simulink model "power_microgrid_v5_battery"  (R2018b)
settings: Solver=ode23tb  StartTime=0.0  StopTime=24*60*60  FixedStep=1/(1000)  MaxStep=60  RelTol=1e-4
PreLoadFcn:
  | load('solar_load_data_24h.mat')
PostLoadFcn:
  | data = xlsread('Domestic_data_all_x3','Sheet1');
  | breakpoints1 = data(2:end,1)'
  | breakpoints2 = data(1,2:end)
  | table_data = data(2:end,2:end)
values from neighbouring files (symbols this model uses):
  SPD_1min = [0 0 0 0 0 0 0 0 0 0 0 0 ... (1441 elements, 1441x1)]    [default_PV_data.mat]
  SPT_1min = [0 60 120 180 240 300 360 420 480 540 600 660 ... (1441 elements, 1441x1)]    [default_PV_data.mat]
libraries: powerlib x155
(part 3 of 5)

== system power_microgrid_v5_battery/House 26 ==
  Clock : Clock
  Complex to Magnitude-Angle : ComplexToMagnitudeAngle  Output=Angle
  Controlled Current Source4 : powerlib/Electrical Sources/Controlled Current Source  Initialize=on  Source_Type=AC  Amplitude=0  Phase=0  Frequency=50  Measurements=None
      settings: SourceProductName=Simscape Electrical
  Gain10 : Gain  Gain=sqrt(2)
  Gain6 : Gain  Gain=-1/230
  Load Data 1-D Lookup Table : Lookup_n-D  NumberOfTableDimensions=1  BreakpointsForDimension1="[0.00\t600.00\t1200.00\t1800.00\t2400.00\t3000.00\t3600.00\t4200.00\t4800.00\t5400.00\t6000.00\t6600.00\t7200.00\t7800.00\t8400.00\t9000.00\t9600.00\t10200.00\t10800.00\t11400.00\t12000.00\t12600.00\t13200.00\t13800.00\t14400.00\t15000.00\t15600.00\t16200.00\t16800.00\t17400.00\t18000.00\t18600.00\t19200.00\t19800.00\t20400.00\t21000.00\t21600.00\t22200.00\t22800.00\t23400.00\t24000.00\t24600.00\t25200.00\t25800.00\t26400.00\t27000.00\t27600.00\t28200.00\t28800.00\t29400.00\t30000.00\t30600.00\t31200.00\t31800.00\t32400.00\t33000.00\t33600.00\t34200.00\t34800.00\t35400.00\t36000.00\t36600.00\t37200.00\t37800.00\t38400.00\t39000.00\t39600.00\t40200.00\t40800.00\t41400.00\t42000.00\t42600.00\t43200.00\t43800.00\t44400.00\t45000.00\t45600.00\t46200.00\t46800.00\t47400.00\t48000.00\t48600.00\t49200.00\t49800.00\t50400.00\t51000.00\t51600.00\t52200.00\t52800.00\t53400.00\t54000.00\t54600.00\t55200.00\t55800.00\t56400.00\t57000.00\t57600.00\t58200.00\t58800.00\t59400.00\t60000.00\t60600.00\t61200.00\t61800.00\t62400.00\t63000.00\t63600.00\t64200.00\t64800.00\t65400.00\t66000.00\t66600.00\t67200.00\t67800.00\t68400.00\t69000.00\t69600.00\t70200.00\t70800.00\t71400.00\t72000.00\t72600.00\t73200.00\t73800.00\t74400.00\t75000.00\t75600.00\t76200.00\t76800.00\t77400.00\t78000.00\t78600.00\t79200.00\t79800.00\t80400.00\t81000.00\t81600.00\t82200.00\t82800.00\t83400.00\t84000.00\t84600.00\t85200.00\t85800.00\t86400.00]"  BeginIndexSearchUsingPreviousIndexResult=on  Table="[176.6\t168.8\t171.0\t162.4\t139.2\t135.7\t136.1\t126.4\t115.3\t119.1\t120.9\t112.9\t108.8\t108.4\t108.6\t115.7\t109.1\t110.1\t104.3\t102.4\t107.1\t108.6\t105.0\t101.7\t101.0\t100.5\t104.1\t105.9\t110.2\t113.1\t112.9\t122.1\t109.2\t120.3\t118.6\t122.6\t124.2\t134.1\t162.8\t189.0\t309.3\t319.3\t364.8\t346.9\t417.0\t276.3\t256.5\t386.4\t343.0\t281.6\t284.9\t297.7\t367.6\t344.5\t340.2\t401.7\t337.5\t290.1\t263.4\t283.0\t256.4\t264.4\t333.9\t339.9\t228.2\t258.4\t286.7\t337.2\t345.7\t283.4\t271.5\t301.9\t315.2\t222.7\t260.5\t314.4\t276.6\t251.0\t286.5\t277.6\t337.1\t293.1\t272.6\t264.0\t234.7\t266.6\t312.4\t300.4\t272.7\t275.3\t328.8\t303.7\t296.9\t271.1\t276.5\t287.6\t336.9\t310.5\t308.1\t352.7\t369.3\t416.5\t395.6\t425.3\t391.6\t343.9\t385.2\t411.7\t419.9\t433.6\t448.9\t437.5\t456.3\t466.2\t475.8\t478.2\t421.9\t455.4\t432.7\t434.7\t414.2\t380.6\t376.3\t380.7\t364.6\t365.6\t376.3\t400.0\t428.4\t382.9\t369.3\t440.8\t388.9\t372.9\t362.3\t328.6\t292.7\t286.7\t266.4\t263.2\t248.0\t239.3\t218.5\t190.8\t176.6]"  InternalRulePriority=Speed  RndMeth=Simplest  InputSameDT=on
  Magnitude-Angle to Complex1 : MagnitudeAngleToComplex
  Snubber3 : powerlib/Elements/Series RLC Branch  LConnTagsString=__new0  RConnTagsString=__new0  BranchType=R  Resistance=1e6  Inductance=1e-3  SetiL0=off  InitialCurrent=0  Capacitance=1e-6  Setx0=off  InitialVoltage=0  Measurements=None
      settings: SourceProductName=Simscape Electrical
  meas cur2 : powerlib/Measurements/Current Measurement  PhasorSimulation=on  OutputType=Complex  PSBequivalent=0
      settings: SourceProductName=Simscape Electrical
  Conn1 : PMIOPort  Side=Left
  Conn2 : PMIOPort  Port=2  Side=Right
  Out1 : Outport
  wires:
  meas cur2/1 -> Out1/1
  Clock/1 -> Load Data 1-D Lookup Table/1
  Magnitude-Angle to Complex1/1 -> Controlled Current Source4/1
  Load Data 1-D Lookup Table/1 -> Gain6/1
  Complex to Magnitude-Angle/1 -> Magnitude-Angle to Complex1/2
  Gain10/1 -> Magnitude-Angle to Complex1/1
  Gain6/1 -> Gain10/1
  [Vsec] -> Complex to Magnitude-Angle/1
  connections:
  Controlled Current Source4/LConn1 -- Conn2/RConn1 -- Snubber3/RConn1
  Controlled Current Source4/RConn1 -- meas cur2/RConn1 -- Snubber3/LConn1
  Conn1/RConn1 -- meas cur2/LConn1

== system power_microgrid_v5_battery/House 27 ==
  Clock : Clock
  Complex to Magnitude-Angle : ComplexToMagnitudeAngle  Output=Angle
  Controlled Current Source4 : powerlib/Electrical Sources/Controlled Current Source  Initialize=on  Source_Type=AC  Amplitude=0  Phase=0  Frequency=50  Measurements=None
      settings: SourceProductName=Simscape Electrical
  Gain10 : Gain  Gain=sqrt(2)
  Gain6 : Gain  Gain=-1/230
  Load Data 1-D Lookup Table : Lookup_n-D  NumberOfTableDimensions=1  BreakpointsForDimension1="[0.00\t600.00\t1200.00\t1800.00\t2400.00\t3000.00\t3600.00\t4200.00\t4800.00\t5400.00\t6000.00\t6600.00\t7200.00\t7800.00\t8400.00\t9000.00\t9600.00\t10200.00\t10800.00\t11400.00\t12000.00\t12600.00\t13200.00\t13800.00\t14400.00\t15000.00\t15600.00\t16200.00\t16800.00\t17400.00\t18000.00\t18600.00\t19200.00\t19800.00\t20400.00\t21000.00\t21600.00\t22200.00\t22800.00\t23400.00\t24000.00\t24600.00\t25200.00\t25800.00\t26400.00\t27000.00\t27600.00\t28200.00\t28800.00\t29400.00\t30000.00\t30600.00\t31200.00\t31800.00\t32400.00\t33000.00\t33600.00\t34200.00\t34800.00\t35400.00\t36000.00\t36600.00\t37200.00\t37800.00\t38400.00\t39000.00\t39600.00\t40200.00\t40800.00\t41400.00\t42000.00\t42600.00\t43200.00\t43800.00\t44400.00\t45000.00\t45600.00\t46200.00\t46800.00\t47400.00\t48000.00\t48600.00\t49200.00\t49800.00\t50400.00\t51000.00\t51600.00\t52200.00\t52800.00\t53400.00\t54000.00\t54600.00\t55200.00\t55800.00\t56400.00\t57000.00\t57600.00\t58200.00\t58800.00\t59400.00\t60000.00\t60600.00\t61200.00\t61800.00\t62400.00\t63000.00\t63600.00\t64200.00\t64800.00\t65400.00\t66000.00\t66600.00\t67200.00\t67800.00\t68400.00\t69000.00\t69600.00\t70200.00\t70800.00\t71400.00\t72000.00\t72600.00\t73200.00\t73800.00\t74400.00\t75000.00\t75600.00\t76200.00\t76800.00\t77400.00\t78000.00\t78600.00\t79200.00\t79800.00\t80400.00\t81000.00\t81600.00\t82200.00\t82800.00\t83400.00\t84000.00\t84600.00\t85200.00\t85800.00\t86400.00]"  BeginIndexSearchUsingPreviousIndexResult=on  Table="[176.6\t168.8\t171.0\t162.4\t139.2\t135.7\t136.1\t126.4\t115.3\t119.1\t120.9\t112.9\t108.8\t108.4\t108.6\t115.7\t109.1\t110.1\t104.3\t102.4\t107.1\t108.6\t105.0\t101.7\t101.0\t100.5\t104.1\t105.9\t110.2\t113.1\t112.9\t122.1\t109.2\t120.3\t118.6\t122.6\t124.2\t134.1\t162.8\t189.0\t309.3\t319.3\t364.8\t346.9\t417.0\t276.3\t256.5\t386.4\t343.0\t281.6\t284.9\t297.7\t367.6\t344.5\t340.2\t401.7\t337.5\t290.1\t263.4\t283.0\t256.4\t264.4\t333.9\t339.9\t228.2\t258.4\t286.7\t337.2\t345.7\t283.4\t271.5\t301.9\t315.2\t222.7\t260.5\t314.4\t276.6\t251.0\t286.5\t277.6\t337.1\t293.1\t272.6\t264.0\t234.7\t266.6\t312.4\t300.4\t272.7\t275.3\t328.8\t303.7\t296.9\t271.1\t276.5\t287.6\t336.9\t310.5\t308.1\t352.7\t369.3\t416.5\t395.6\t425.3\t391.6\t343.9\t385.2\t411.7\t419.9\t433.6\t448.9\t437.5\t456.3\t466.2\t475.8\t478.2\t421.9\t455.4\t432.7\t434.7\t414.2\t380.6\t376.3\t380.7\t364.6\t365.6\t376.3\t400.0\t428.4\t382.9\t369.3\t440.8\t388.9\t372.9\t362.3\t328.6\t292.7\t286.7\t266.4\t263.2\t248.0\t239.3\t218.5\t190.8\t176.6]"  InternalRulePriority=Speed  RndMeth=Simplest  InputSameDT=on
  Magnitude-Angle to Complex1 : MagnitudeAngleToComplex
  Snubber3 : powerlib/Elements/Series RLC Branch  LConnTagsString=__new0  RConnTagsString=__new0  BranchType=R  Resistance=1e6  Inductance=1e-3  SetiL0=off  InitialCurrent=0  Capacitance=1e-6  Setx0=off  InitialVoltage=0  Measurements=None
      settings: SourceProductName=Simscape Electrical
  meas cur2 : powerlib/Measurements/Current Measurement  PhasorSimulation=on  OutputType=Complex  PSBequivalent=0
      settings: SourceProductName=Simscape Electrical
  Conn1 : PMIOPort  Side=Left
  Conn2 : PMIOPort  Port=2  Side=Right
  Out1 : Outport
  wires:
  meas cur2/1 -> Out1/1
  Clock/1 -> Load Data 1-D Lookup Table/1
  Magnitude-Angle to Complex1/1 -> Controlled Current Source4/1
  Load Data 1-D Lookup Table/1 -> Gain6/1
  Complex to Magnitude-Angle/1 -> Magnitude-Angle to Complex1/2
  Gain10/1 -> Magnitude-Angle to Complex1/1
  Gain6/1 -> Gain10/1
  [Vsec] -> Complex to Magnitude-Angle/1
  connections:
  Conn1/RConn1 -- meas cur2/LConn1
  Snubber3/LConn1 -- meas cur2/RConn1 -- Controlled Current Source4/RConn1
  Snubber3/RConn1 -- Controlled Current Source4/LConn1 -- Conn2/RConn1

== system power_microgrid_v5_battery/House 28 ==
  Clock : Clock
  Complex to Magnitude-Angle : ComplexToMagnitudeAngle  Output=Angle
  Controlled Current Source4 : powerlib/Electrical Sources/Controlled Current Source  Initialize=on  Source_Type=AC  Amplitude=0  Phase=0  Frequency=50  Measurements=None
      settings: SourceProductName=Simscape Electrical
  Gain10 : Gain  Gain=sqrt(2)
  Gain6 : Gain  Gain=-1/230
  Load Data 1-D Lookup Table : Lookup_n-D  NumberOfTableDimensions=1  BreakpointsForDimension1="[0.00\t600.00\t1200.00\t1800.00\t2400.00\t3000.00\t3600.00\t4200.00\t4800.00\t5400.00\t6000.00\t6600.00\t7200.00\t7800.00\t8400.00\t9000.00\t9600.00\t10200.00\t10800.00\t11400.00\t12000.00\t12600.00\t13200.00\t13800.00\t14400.00\t15000.00\t15600.00\t16200.00\t16800.00\t17400.00\t18000.00\t18600.00\t19200.00\t19800.00\t20400.00\t21000.00\t21600.00\t22200.00\t22800.00\t23400.00\t24000.00\t24600.00\t25200.00\t25800.00\t26400.00\t27000.00\t27600.00\t28200.00\t28800.00\t29400.00\t30000.00\t30600.00\t31200.00\t31800.00\t32400.00\t33000.00\t33600.00\t34200.00\t34800.00\t35400.00\t36000.00\t36600.00\t37200.00\t37800.00\t38400.00\t39000.00\t39600.00\t40200.00\t40800.00\t41400.00\t42000.00\t42600.00\t43200.00\t43800.00\t44400.00\t45000.00\t45600.00\t46200.00\t46800.00\t47400.00\t48000.00\t48600.00\t49200.00\t49800.00\t50400.00\t51000.00\t51600.00\t52200.00\t52800.00\t53400.00\t54000.00\t54600.00\t55200.00\t55800.00\t56400.00\t57000.00\t57600.00\t58200.00\t58800.00\t59400.00\t60000.00\t60600.00\t61200.00\t61800.00\t62400.00\t63000.00\t63600.00\t64200.00\t64800.00\t65400.00\t66000.00\t66600.00\t67200.00\t67800.00\t68400.00\t69000.00\t69600.00\t70200.00\t70800.00\t71400.00\t72000.00\t72600.00\t73200.00\t73800.00\t74400.00\t75000.00\t75600.00\t76200.00\t76800.00\t77400.00\t78000.00\t78600.00\t79200.00\t79800.00\t80400.00\t81000.00\t81600.00\t82200.00\t82800.00\t83400.00\t84000.00\t84600.00\t85200.00\t85800.00\t86400.00]"  BeginIndexSearchUsingPreviousIndexResult=on  Table="[176.6\t168.8\t171.0\t162.4\t139.2\t135.7\t136.1\t126.4\t115.3\t119.1\t120.9\t112.9\t108.8\t108.4\t108.6\t115.7\t109.1\t110.1\t104.3\t102.4\t107.1\t108.6\t105.0\t101.7\t101.0\t100.5\t104.1\t105.9\t110.2\t113.1\t112.9\t122.1\t109.2\t120.3\t118.6\t122.6\t124.2\t134.1\t162.8\t189.0\t309.3\t319.3\t364.8\t346.9\t417.0\t276.3\t256.5\t386.4\t343.0\t281.6\t284.9\t297.7\t367.6\t344.5\t340.2\t401.7\t337.5\t290.1\t263.4\t283.0\t256.4\t264.4\t333.9\t339.9\t228.2\t258.4\t286.7\t337.2\t345.7\t283.4\t271.5\t301.9\t315.2\t222.7\t260.5\t314.4\t276.6\t251.0\t286.5\t277.6\t337.1\t293.1\t272.6\t264.0\t234.7\t266.6\t312.4\t300.4\t272.7\t275.3\t328.8\t303.7\t296.9\t271.1\t276.5\t287.6\t336.9\t310.5\t308.1\t352.7\t369.3\t416.5\t395.6\t425.3\t391.6\t343.9\t385.2\t411.7\t419.9\t433.6\t448.9\t437.5\t456.3\t466.2\t475.8\t478.2\t421.9\t455.4\t432.7\t434.7\t414.2\t380.6\t376.3\t380.7\t364.6\t365.6\t376.3\t400.0\t428.4\t382.9\t369.3\t440.8\t388.9\t372.9\t362.3\t328.6\t292.7\t286.7\t266.4\t263.2\t248.0\t239.3\t218.5\t190.8\t176.6]"  InternalRulePriority=Speed  RndMeth=Simplest  InputSameDT=on
  Magnitude-Angle to Complex1 : MagnitudeAngleToComplex
  Snubber3 : powerlib/Elements/Series RLC Branch  LConnTagsString=__new0  RConnTagsString=__new0  BranchType=R  Resistance=1e6  Inductance=1e-3  SetiL0=off  InitialCurrent=0  Capacitance=1e-6  Setx0=off  InitialVoltage=0  Measurements=None
      settings: SourceProductName=Simscape Electrical
  meas cur2 : powerlib/Measurements/Current Measurement  PhasorSimulation=on  OutputType=Complex  PSBequivalent=0
      settings: SourceProductName=Simscape Electrical
  Conn1 : PMIOPort  Side=Left
  Conn2 : PMIOPort  Port=2  Side=Right
  Out1 : Outport
  wires:
  meas cur2/1 -> Out1/1
  Clock/1 -> Load Data 1-D Lookup Table/1
  Magnitude-Angle to Complex1/1 -> Controlled Current Source4/1
  Load Data 1-D Lookup Table/1 -> Gain6/1
  Complex to Magnitude-Angle/1 -> Magnitude-Angle to Complex1/2
  Gain10/1 -> Magnitude-Angle to Complex1/1
  Gain6/1 -> Gain10/1
  [Vsec] -> Complex to Magnitude-Angle/1
  connections:
  Conn1/RConn1 -- meas cur2/LConn1
  Snubber3/LConn1 -- meas cur2/RConn1 -- Controlled Current Source4/RConn1
  Snubber3/RConn1 -- Controlled Current Source4/LConn1 -- Conn2/RConn1

== system power_microgrid_v5_battery/House 29 ==
  Clock : Clock
  Complex to Magnitude-Angle : ComplexToMagnitudeAngle  Output=Angle
  Controlled Current Source4 : powerlib/Electrical Sources/Controlled Current Source  Initialize=on  Source_Type=AC  Amplitude=0  Phase=0  Frequency=50  Measurements=None
      settings: SourceProductName=Simscape Electrical
  Gain10 : Gain  Gain=sqrt(2)
  Gain6 : Gain  Gain=-1/230
  Load Data 1-D Lookup Table : Lookup_n-D  NumberOfTableDimensions=1  BreakpointsForDimension1="[0.00\t600.00\t1200.00\t1800.00\t2400.00\t3000.00\t3600.00\t4200.00\t4800.00\t5400.00\t6000.00\t6600.00\t7200.00\t7800.00\t8400.00\t9000.00\t9600.00\t10200.00\t10800.00\t11400.00\t12000.00\t12600.00\t13200.00\t13800.00\t14400.00\t15000.00\t15600.00\t16200.00\t16800.00\t17400.00\t18000.00\t18600.00\t19200.00\t19800.00\t20400.00\t21000.00\t21600.00\t22200.00\t22800.00\t23400.00\t24000.00\t24600.00\t25200.00\t25800.00\t26400.00\t27000.00\t27600.00\t28200.00\t28800.00\t29400.00\t30000.00\t30600.00\t31200.00\t31800.00\t32400.00\t33000.00\t33600.00\t34200.00\t34800.00\t35400.00\t36000.00\t36600.00\t37200.00\t37800.00\t38400.00\t39000.00\t39600.00\t40200.00\t40800.00\t41400.00\t42000.00\t42600.00\t43200.00\t43800.00\t44400.00\t45000.00\t45600.00\t46200.00\t46800.00\t47400.00\t48000.00\t48600.00\t49200.00\t49800.00\t50400.00\t51000.00\t51600.00\t52200.00\t52800.00\t53400.00\t54000.00\t54600.00\t55200.00\t55800.00\t56400.00\t57000.00\t57600.00\t58200.00\t58800.00\t59400.00\t60000.00\t60600.00\t61200.00\t61800.00\t62400.00\t63000.00\t63600.00\t64200.00\t64800.00\t65400.00\t66000.00\t66600.00\t67200.00\t67800.00\t68400.00\t69000.00\t69600.00\t70200.00\t70800.00\t71400.00\t72000.00\t72600.00\t73200.00\t73800.00\t74400.00\t75000.00\t75600.00\t76200.00\t76800.00\t77400.00\t78000.00\t78600.00\t79200.00\t79800.00\t80400.00\t81000.00\t81600.00\t82200.00\t82800.00\t83400.00\t84000.00\t84600.00\t85200.00\t85800.00\t86400.00]"  BeginIndexSearchUsingPreviousIndexResult=on  Table="[176.6\t168.8\t171.0\t162.4\t139.2\t135.7\t136.1\t126.4\t115.3\t119.1\t120.9\t112.9\t108.8\t108.4\t108.6\t115.7\t109.1\t110.1\t104.3\t102.4\t107.1\t108.6\t105.0\t101.7\t101.0\t100.5\t104.1\t105.9\t110.2\t113.1\t112.9\t122.1\t109.2\t120.3\t118.6\t122.6\t124.2\t134.1\t162.8\t189.0\t309.3\t319.3\t364.8\t346.9\t417.0\t276.3\t256.5\t386.4\t343.0\t281.6\t284.9\t297.7\t367.6\t344.5\t340.2\t401.7\t337.5\t290.1\t263.4\t283.0\t256.4\t264.4\t333.9\t339.9\t228.2\t258.4\t286.7\t337.2\t345.7\t283.4\t271.5\t301.9\t315.2\t222.7\t260.5\t314.4\t276.6\t251.0\t286.5\t277.6\t337.1\t293.1\t272.6\t264.0\t234.7\t266.6\t312.4\t300.4\t272.7\t275.3\t328.8\t303.7\t296.9\t271.1\t276.5\t287.6\t336.9\t310.5\t308.1\t352.7\t369.3\t416.5\t395.6\t425.3\t391.6\t343.9\t385.2\t411.7\t419.9\t433.6\t448.9\t437.5\t456.3\t466.2\t475.8\t478.2\t421.9\t455.4\t432.7\t434.7\t414.2\t380.6\t376.3\t380.7\t364.6\t365.6\t376.3\t400.0\t428.4\t382.9\t369.3\t440.8\t388.9\t372.9\t362.3\t328.6\t292.7\t286.7\t266.4\t263.2\t248.0\t239.3\t218.5\t190.8\t176.6]"  InternalRulePriority=Speed  RndMeth=Simplest  InputSameDT=on
  Magnitude-Angle to Complex1 : MagnitudeAngleToComplex
  Snubber3 : powerlib/Elements/Series RLC Branch  LConnTagsString=__new0  RConnTagsString=__new0  BranchType=R  Resistance=1e6  Inductance=1e-3  SetiL0=off  InitialCurrent=0  Capacitance=1e-6  Setx0=off  InitialVoltage=0  Measurements=None
      settings: SourceProductName=Simscape Electrical
  meas cur2 : powerlib/Measurements/Current Measurement  PhasorSimulation=on  OutputType=Complex  PSBequivalent=0
      settings: SourceProductName=Simscape Electrical
  Conn1 : PMIOPort  Side=Left
  Conn2 : PMIOPort  Port=2  Side=Right
  Out1 : Outport
  wires:
  meas cur2/1 -> Out1/1
  Clock/1 -> Load Data 1-D Lookup Table/1
  Magnitude-Angle to Complex1/1 -> Controlled Current Source4/1
  Load Data 1-D Lookup Table/1 -> Gain6/1
  Complex to Magnitude-Angle/1 -> Magnitude-Angle to Complex1/2
  Gain10/1 -> Magnitude-Angle to Complex1/1
  Gain6/1 -> Gain10/1
  [Vsec] -> Complex to Magnitude-Angle/1
  connections:
  Conn1/RConn1 -- meas cur2/LConn1
  Snubber3/LConn1 -- meas cur2/RConn1 -- Controlled Current Source4/RConn1
  Snubber3/RConn1 -- Controlled Current Source4/LConn1 -- Conn2/RConn1

== system power_microgrid_v5_battery/House 3 ==
  Clock : Clock
  Complex to Magnitude-Angle : ComplexToMagnitudeAngle  Output=Angle
  Controlled Current Source4 : powerlib/Electrical Sources/Controlled Current Source  Initialize=on  Source_Type=AC  Amplitude=0  Phase=0  Frequency=50  Measurements=None
      settings: SourceProductName=Simscape Electrical
  Gain10 : Gain  Gain=sqrt(2)
  Gain6 : Gain  Gain=-1/230
  Load Data 1-D Lookup Table : Lookup_n-D  NumberOfTableDimensions=1  BreakpointsForDimension1="[0.00\t600.00\t1200.00\t1800.00\t2400.00\t3000.00\t3600.00\t4200.00\t4800.00\t5400.00\t6000.00\t6600.00\t7200.00\t7800.00\t8400.00\t9000.00\t9600.00\t10200.00\t10800.00\t11400.00\t12000.00\t12600.00\t13200.00\t13800.00\t14400.00\t15000.00\t15600.00\t16200.00\t16800.00\t17400.00\t18000.00\t18600.00\t19200.00\t19800.00\t20400.00\t21000.00\t21600.00\t22200.00\t22800.00\t23400.00\t24000.00\t24600.00\t25200.00\t25800.00\t26400.00\t27000.00\t27600.00\t28200.00\t28800.00\t29400.00\t30000.00\t30600.00\t31200.00\t31800.00\t32400.00\t33000.00\t33600.00\t34200.00\t34800.00\t35400.00\t36000.00\t36600.00\t37200.00\t37800.00\t38400.00\t39000.00\t39600.00\t40200.00\t40800.00\t41400.00\t42000.00\t42600.00\t43200.00\t43800.00\t44400.00\t45000.00\t45600.00\t46200.00\t46800.00\t47400.00\t48000.00\t48600.00\t49200.00\t49800.00\t50400.00\t51000.00\t51600.00\t52200.00\t52800.00\t53400.00\t54000.00\t54600.00\t55200.00\t55800.00\t56400.00\t57000.00\t57600.00\t58200.00\t58800.00\t59400.00\t60000.00\t60600.00\t61200.00\t61800.00\t62400.00\t63000.00\t63600.00\t64200.00\t64800.00\t65400.00\t66000.00\t66600.00\t67200.00\t67800.00\t68400.00\t69000.00\t69600.00\t70200.00\t70800.00\t71400.00\t72000.00\t72600.00\t73200.00\t73800.00\t74400.00\t75000.00\t75600.00\t76200.00\t76800.00\t77400.00\t78000.00\t78600.00\t79200.00\t79800.00\t80400.00\t81000.00\t81600.00\t82200.00\t82800.00\t83400.00\t84000.00\t84600.00\t85200.00\t85800.00\t86400.00]"  BeginIndexSearchUsingPreviousIndexResult=on  Table="[179.5\t163.3\t152.9\t132.5\t118.9\t111.3\t124.6\t103.3\t83.5\t81.2\t85.9\t85.2\t91.9\t95.6\t95.9\t81.8\t83.7\t86.7\t93.8\t81.2\t92.7\t99.4\t112.6\t88.2\t85.6\t78.4\t88.4\t93.9\t86.1\t86.0\t111.7\t143.5\t122.7\t136.8\t142.2\t135.1\t145.6\t141.8\t152.1\t140.3\t167.9\t256.6\t226.1\t263.8\t283.9\t303.3\t279.5\t294.9\t282.3\t288.8\t333.5\t360.9\t421.4\t494.2\t392.5\t439.7\t395.9\t394.4\t364.9\t353.0\t359.1\t370.9\t398.5\t447.4\t344.5\t330.8\t306.8\t331.3\t331.9\t307.6\t371.3\t387.4\t376.6\t360.2\t414.1\t445.1\t411.1\t389.5\t425.2\t340.0\t316.3\t332.8\t352.3\t301.8\t261.8\t298.1\t350.9\t327.8\t296.5\t319.6\t368.4\t327.2\t265.7\t277.9\t292.9\t301.4\t377.9\t336.0\t324.6\t353.8\t389.7\t355.9\t328.4\t325.9\t378.1\t338.0\t379.1\t414.8\t418.1\t464.8\t488.1\t489.1\t485.7\t581.3\t579.7\t526.2\t551.4\t618.6\t628.5\t578.8\t553.3\t481.5\t455.6\t487.9\t507.3\t497.6\t515.4\t510.2\t490.5\t500.5\t494.1\t532.9\t506.5\t466.6\t438.0\t385.4\t381.2\t385.9\t351.7\t371.3\t340.8\t320.2\t277.0\t228.9\t179.5]"  InternalRulePriority=Speed  RndMeth=Simplest  InputSameDT=on
  Magnitude-Angle to Complex1 : MagnitudeAngleToComplex
  Snubber3 : powerlib/Elements/Series RLC Branch  LConnTagsString=__new0  RConnTagsString=__new0  BranchType=R  Resistance=1e6  Inductance=1e-3  SetiL0=off  InitialCurrent=0  Capacitance=1e-6  Setx0=off  InitialVoltage=0  Measurements=None
      settings: SourceProductName=Simscape Electrical
  meas cur2 : powerlib/Measurements/Current Measurement  PhasorSimulation=on  OutputType=Complex  PSBequivalent=0
      settings: SourceProductName=Simscape Electrical
  Conn1 : PMIOPort  Side=Left
  Conn2 : PMIOPort  Port=2  Side=Right
  Out1 : Outport
  wires:
  meas cur2/1 -> Out1/1
  Clock/1 -> Load Data 1-D Lookup Table/1
  Magnitude-Angle to Complex1/1 -> Controlled Current Source4/1
  Load Data 1-D Lookup Table/1 -> Gain6/1
  Complex to Magnitude-Angle/1 -> Magnitude-Angle to Complex1/2
  Gain10/1 -> Magnitude-Angle to Complex1/1
  Gain6/1 -> Gain10/1
  [Vsec] -> Complex to Magnitude-Angle/1
  connections:
  Conn1/RConn1 -- meas cur2/LConn1
  Snubber3/LConn1 -- meas cur2/RConn1 -- Controlled Current Source4/RConn1
  Snubber3/RConn1 -- Controlled Current Source4/LConn1 -- Conn2/RConn1

== system power_microgrid_v5_battery/House 31 ==
  Clock : Clock
  Complex to Magnitude-Angle : ComplexToMagnitudeAngle  Output=Angle
  Controlled Current Source4 : powerlib/Electrical Sources/Controlled Current Source  Initialize=on  Source_Type=AC  Amplitude=0  Phase=0  Frequency=50  Measurements=None
      settings: SourceProductName=Simscape Electrical
  Gain10 : Gain  Gain=sqrt(2)
  Gain6 : Gain  Gain=-1/230
  Load Data 1-D Lookup Table : Lookup_n-D  NumberOfTableDimensions=1  BreakpointsForDimension1="[0.00\t600.00\t1200.00\t1800.00\t2400.00\t3000.00\t3600.00\t4200.00\t4800.00\t5400.00\t6000.00\t6600.00\t7200.00\t7800.00\t8400.00\t9000.00\t9600.00\t10200.00\t10800.00\t11400.00\t12000.00\t12600.00\t13200.00\t13800.00\t14400.00\t15000.00\t15600.00\t16200.00\t16800.00\t17400.00\t18000.00\t18600.00\t19200.00\t19800.00\t20400.00\t21000.00\t21600.00\t22200.00\t22800.00\t23400.00\t24000.00\t24600.00\t25200.00\t25800.00\t26400.00\t27000.00\t27600.00\t28200.00\t28800.00\t29400.00\t30000.00\t30600.00\t31200.00\t31800.00\t32400.00\t33000.00\t33600.00\t34200.00\t34800.00\t35400.00\t36000.00\t36600.00\t37200.00\t37800.00\t38400.00\t39000.00\t39600.00\t40200.00\t40800.00\t41400.00\t42000.00\t42600.00\t43200.00\t43800.00\t44400.00\t45000.00\t45600.00\t46200.00\t46800.00\t47400.00\t48000.00\t48600.00\t49200.00\t49800.00\t50400.00\t51000.00\t51600.00\t52200.00\t52800.00\t53400.00\t54000.00\t54600.00\t55200.00\t55800.00\t56400.00\t57000.00\t57600.00\t58200.00\t58800.00\t59400.00\t60000.00\t60600.00\t61200.00\t61800.00\t62400.00\t63000.00\t63600.00\t64200.00\t64800.00\t65400.00\t66000.00\t66600.00\t67200.00\t67800.00\t68400.00\t69000.00\t69600.00\t70200.00\t70800.00\t71400.00\t72000.00\t72600.00\t73200.00\t73800.00\t74400.00\t75000.00\t75600.00\t76200.00\t76800.00\t77400.00\t78000.00\t78600.00\t79200.00\t79800.00\t80400.00\t81000.00\t81600.00\t82200.00\t82800.00\t83400.00\t84000.00\t84600.00\t85200.00\t85800.00\t86400.00]"  BeginIndexSearchUsingPreviousIndexResult=on  Table="[274.3\t264.8\t264.4\t270.0\t249.7\t231.6\t207.3\t346.0\t405.4\t427.1\t427.7\t390.1\t362.8\t323.2\t235.2\t200.1\t175.7\t182.2\t191.8\t179.5\t176.0\t191.1\t182.4\t189.5\t381.6\t362.5\t360.8\t259.0\t236.4\t190.9\t185.6\t202.5\t180.1\t171.6\t178.6\t205.5\t197.7\t204.6\t268.7\t226.2\t283.1\t267.9\t263.1\t273.4\t310.8\t342.7\t324.3\t374.3\t479.4\t468.8\t413.5\t422.8\t407.2\t385.7\t388.9\t466.4\t498.9\t472.2\t410.3\t402.7\t401.3\t393.2\t428.4\t409.0\t366.8\t363.8\t350.9\t379.0\t491.1\t424.1\t418.6\t424.3\t381.3\t396.5\t350.9\t334.4\t302.5\t322.4\t363.2\t434.6\t394.2\t382.2\t385.1\t366.7\t349.4\t326.2\t305.1\t309.1\t308.8\t317.1\t343.5\t377.4\t366.8\t381.4\t390.3\t399.4\t414.2\t461.9\t415.5\t442.2\t453.9\t501.6\t488.3\t480.3\t508.6\t522.0\t476.2\t559.6\t510.9\t522.6\t506.1\t515.6\t527.0\t554.7\t515.5\t523.0\t525.4\t514.0\t492.4\t498.0\t460.9\t521.0\t480.2\t477.2\t455.1\t449.4\t459.8\t475.1\t457.6\t484.0\t474.3\t440.2\t421.1\t436.3\t435.7\t385.1\t385.1\t362.9\t360.9\t327.6\t315.6\t294.6\t290.2\t275.5\t274.3]"  InternalRulePriority=Speed  RndMeth=Simplest  InputSameDT=on
  Magnitude-Angle to Complex1 : MagnitudeAngleToComplex
  Snubber3 : powerlib/Elements/Series RLC Branch  LConnTagsString=__new0  RConnTagsString=__new0  BranchType=R  Resistance=1e6  Inductance=1e-3  SetiL0=off  InitialCurrent=0  Capacitance=1e-6  Setx0=off  InitialVoltage=0  Measurements=None
      settings: SourceProductName=Simscape Electrical
  meas cur2 : powerlib/Measurements/Current Measurement  PhasorSimulation=on  OutputType=Complex  PSBequivalent=0
      settings: SourceProductName=Simscape Electrical
  Conn1 : PMIOPort  Side=Left
  Conn2 : PMIOPort  Port=2  Side=Right
  Out1 : Outport
  wires:
  Magnitude-Angle to Complex1/1 -> Controlled Current Source4/1
  meas cur2/1 -> Out1/1
  Clock/1 -> Load Data 1-D Lookup Table/1
  Load Data 1-D Lookup Table/1 -> Gain6/1
  [Vsec] -> Complex to Magnitude-Angle/1
  Gain6/1 -> Gain10/1
  Gain10/1 -> Magnitude-Angle to Complex1/1
  Complex to Magnitude-Angle/1 -> Magnitude-Angle to Complex1/2
  connections:
  meas cur2/LConn1 -- Conn1/RConn1
  Snubber3/LConn1 -- Controlled Current Source4/RConn1 -- meas cur2/RConn1
  Snubber3/RConn1 -- Controlled Current Source4/LConn1 -- Conn2/RConn1

== system power_microgrid_v5_battery/House 32 ==
  Clock : Clock
  Complex to Magnitude-Angle : ComplexToMagnitudeAngle  Output=Angle
  Controlled Current Source4 : powerlib/Electrical Sources/Controlled Current Source  Initialize=on  Source_Type=AC  Amplitude=0  Phase=0  Frequency=50  Measurements=None
      settings: SourceProductName=Simscape Electrical
  Gain10 : Gain  Gain=sqrt(2)
  Gain6 : Gain  Gain=-1/230
  Load Data 1-D Lookup Table : Lookup_n-D  NumberOfTableDimensions=1  BreakpointsForDimension1="[0.00\t600.00\t1200.00\t1800.00\t2400.00\t3000.00\t3600.00\t4200.00\t4800.00\t5400.00\t6000.00\t6600.00\t7200.00\t7800.00\t8400.00\t9000.00\t9600.00\t10200.00\t10800.00\t11400.00\t12000.00\t12600.00\t13200.00\t13800.00\t14400.00\t15000.00\t15600.00\t16200.00\t16800.00\t17400.00\t18000.00\t18600.00\t19200.00\t19800.00\t20400.00\t21000.00\t21600.00\t22200.00\t22800.00\t23400.00\t24000.00\t24600.00\t25200.00\t25800.00\t26400.00\t27000.00\t27600.00\t28200.00\t28800.00\t29400.00\t30000.00\t30600.00\t31200.00\t31800.00\t32400.00\t33000.00\t33600.00\t34200.00\t34800.00\t35400.00\t36000.00\t36600.00\t37200.00\t37800.00\t38400.00\t39000.00\t39600.00\t40200.00\t40800.00\t41400.00\t42000.00\t42600.00\t43200.00\t43800.00\t44400.00\t45000.00\t45600.00\t46200.00\t46800.00\t47400.00\t48000.00\t48600.00\t49200.00\t49800.00\t50400.00\t51000.00\t51600.00\t52200.00\t52800.00\t53400.00\t54000.00\t54600.00\t55200.00\t55800.00\t56400.00\t57000.00\t57600.00\t58200.00\t58800.00\t59400.00\t60000.00\t60600.00\t61200.00\t61800.00\t62400.00\t63000.00\t63600.00\t64200.00\t64800.00\t65400.00\t66000.00\t66600.00\t67200.00\t67800.00\t68400.00\t69000.00\t69600.00\t70200.00\t70800.00\t71400.00\t72000.00\t72600.00\t73200.00\t73800.00\t74400.00\t75000.00\t75600.00\t76200.00\t76800.00\t77400.00\t78000.00\t78600.00\t79200.00\t79800.00\t80400.00\t81000.00\t81600.00\t82200.00\t82800.00\t83400.00\t84000.00\t84600.00\t85200.00\t85800.00\t86400.00]"  BeginIndexSearchUsingPreviousIndexResult=on  Table="[239.5\t239.3\t230.7\t221.1\t236.7\t224.0\t212.7\t208.1\t198.4\t189.5\t188.5\t190.5\t188.9\t175.4\t181.1\t172.1\t176.3\t181.6\t168.9\t165.2\t160.0\t171.7\t173.3\t158.7\t161.2\t183.5\t182.5\t185.8\t174.7\t172.1\t172.3\t171.8\t196.0\t196.8\t185.5\t191.4\t195.5\t211.1\t225.6\t240.9\t294.0\t327.5\t322.1\t404.9\t489.6\t440.2\t382.2\t398.2\t392.8\t423.0\t511.9\t472.7\t420.5\t405.4\t368.1\t353.8\t392.6\t414.0\t406.8\t409.2\t418.6\t483.6\t444.8\t421.6\t429.0\t444.4\t466.1\t457.6\t477.5\t422.1\t438.5\t445.5\t481.4\t506.4\t471.7\t425.1\t441.5\t411.9\t413.0\t436.9\t429.4\t446.6\t455.6\t465.0\t461.5\t475.0\t453.6\t447.1\t473.5\t480.7\t494.8\t468.2\t491.4\t470.2\t471.6\t525.4\t540.8\t554.3\t565.1\t626.5\t743.4\t744.6\t717.5\t733.8\t778.9\t822.7\t807.8\t820.4\t832.5\t863.5\t825.7\t764.6\t774.5\t717.8\t709.4\t778.0\t738.5\t753.7\t739.0\t770.0\t756.2\t812.2\t746.3\t716.1\t705.9\t737.2\t679.1\t623.3\t583.2\t563.0\t523.2\t504.6\t460.7\t440.9\t392.2\t372.0\t362.3\t339.5\t315.3\t289.8\t274.7\t275.1\t266.0\t264.5\t239.5]"  InternalRulePriority=Speed  RndMeth=Simplest  InputSameDT=on
  Magnitude-Angle to Complex1 : MagnitudeAngleToComplex
  Snubber3 : powerlib/Elements/Series RLC Branch  LConnTagsString=__new0  RConnTagsString=__new0  BranchType=R  Resistance=1e6  Inductance=1e-3  SetiL0=off  InitialCurrent=0  Capacitance=1e-6  Setx0=off  InitialVoltage=0  Measurements=None
      settings: SourceProductName=Simscape Electrical
  meas cur2 : powerlib/Measurements/Current Measurement  PhasorSimulation=on  OutputType=Complex  PSBequivalent=0
      settings: SourceProductName=Simscape Electrical
  Conn1 : PMIOPort  Side=Left
  Conn2 : PMIOPort  Port=2  Side=Right
  Out1 : Outport
  wires:
  meas cur2/1 -> Out1/1
  Clock/1 -> Load Data 1-D Lookup Table/1
  Magnitude-Angle to Complex1/1 -> Controlled Current Source4/1
  Load Data 1-D Lookup Table/1 -> Gain6/1
  Complex to Magnitude-Angle/1 -> Magnitude-Angle to Complex1/2
  Gain10/1 -> Magnitude-Angle to Complex1/1
  Gain6/1 -> Gain10/1
  [Vsec] -> Complex to Magnitude-Angle/1
  connections:
  Conn1/RConn1 -- meas cur2/LConn1
  Snubber3/LConn1 -- meas cur2/RConn1 -- Controlled Current Source4/RConn1
  Snubber3/RConn1 -- Controlled Current Source4/LConn1 -- Conn2/RConn1

== system power_microgrid_v5_battery/House 33 ==
  Clock : Clock
  Complex to Magnitude-Angle : ComplexToMagnitudeAngle  Output=Angle
  Controlled Current Source4 : powerlib/Electrical Sources/Controlled Current Source  Initialize=on  Source_Type=AC  Amplitude=0  Phase=0  Frequency=50  Measurements=None
      settings: SourceProductName=Simscape Electrical
  Gain10 : Gain  Gain=sqrt(2)
  Gain6 : Gain  Gain=-1/230
  Load Data 1-D Lookup Table : Lookup_n-D  NumberOfTableDimensions=1  BreakpointsForDimension1="[0.00\t600.00\t1200.00\t1800.00\t2400.00\t3000.00\t3600.00\t4200.00\t4800.00\t5400.00\t6000.00\t6600.00\t7200.00\t7800.00\t8400.00\t9000.00\t9600.00\t10200.00\t10800.00\t11400.00\t12000.00\t12600.00\t13200.00\t13800.00\t14400.00\t15000.00\t15600.00\t16200.00\t16800.00\t17400.00\t18000.00\t18600.00\t19200.00\t19800.00\t20400.00\t21000.00\t21600.00\t22200.00\t22800.00\t23400.00\t24000.00\t24600.00\t25200.00\t25800.00\t26400.00\t27000.00\t27600.00\t28200.00\t28800.00\t29400.00\t30000.00\t30600.00\t31200.00\t31800.00\t32400.00\t33000.00\t33600.00\t34200.00\t34800.00\t35400.00\t36000.00\t36600.00\t37200.00\t37800.00\t38400.00\t39000.00\t39600.00\t40200.00\t40800.00\t41400.00\t42000.00\t42600.00\t43200.00\t43800.00\t44400.00\t45000.00\t45600.00\t46200.00\t46800.00\t47400.00\t48000.00\t48600.00\t49200.00\t49800.00\t50400.00\t51000.00\t51600.00\t52200.00\t52800.00\t53400.00\t54000.00\t54600.00\t55200.00\t55800.00\t56400.00\t57000.00\t57600.00\t58200.00\t58800.00\t59400.00\t60000.00\t60600.00\t61200.00\t61800.00\t62400.00\t63000.00\t63600.00\t64200.00\t64800.00\t65400.00\t66000.00\t66600.00\t67200.00\t67800.00\t68400.00\t69000.00\t69600.00\t70200.00\t70800.00\t71400.00\t72000.00\t72600.00\t73200.00\t73800.00\t74400.00\t75000.00\t75600.00\t76200.00\t76800.00\t77400.00\t78000.00\t78600.00\t79200.00\t79800.00\t80400.00\t81000.00\t81600.00\t82200.00\t82800.00\t83400.00\t84000.00\t84600.00\t85200.00\t85800.00\t86400.00]"  BeginIndexSearchUsingPreviousIndexResult=on  Table="[274.3\t264.8\t264.4\t270.0\t249.7\t231.6\t207.3\t346.0\t405.4\t427.1\t427.7\t390.1\t362.8\t323.2\t235.2\t200.1\t175.7\t182.2\t191.8\t179.5\t176.0\t191.1\t182.4\t189.5\t381.6\t362.5\t360.8\t259.0\t236.4\t190.9\t185.6\t202.5\t180.1\t171.6\t178.6\t205.5\t197.7\t204.6\t268.7\t226.2\t283.1\t267.9\t263.1\t273.4\t310.8\t342.7\t324.3\t374.3\t479.4\t468.8\t413.5\t422.8\t407.2\t385.7\t388.9\t466.4\t498.9\t472.2\t410.3\t402.7\t401.3\t393.2\t428.4\t409.0\t366.8\t363.8\t350.9\t379.0\t491.1\t424.1\t418.6\t424.3\t381.3\t396.5\t350.9\t334.4\t302.5\t322.4\t363.2\t434.6\t394.2\t382.2\t385.1\t366.7\t349.4\t326.2\t305.1\t309.1\t308.8\t317.1\t343.5\t377.4\t366.8\t381.4\t390.3\t399.4\t414.2\t461.9\t415.5\t442.2\t453.9\t501.6\t488.3\t480.3\t508.6\t522.0\t476.2\t559.6\t510.9\t522.6\t506.1\t515.6\t527.0\t554.7\t515.5\t523.0\t525.4\t514.0\t492.4\t498.0\t460.9\t521.0\t480.2\t477.2\t455.1\t449.4\t459.8\t475.1\t457.6\t484.0\t474.3\t440.2\t421.1\t436.3\t435.7\t385.1\t385.1\t362.9\t360.9\t327.6\t315.6\t294.6\t290.2\t275.5\t274.3]"  InternalRulePriority=Speed  RndMeth=Simplest  InputSameDT=on
  Magnitude-Angle to Complex1 : MagnitudeAngleToComplex
  Snubber3 : powerlib/Elements/Series RLC Branch  LConnTagsString=__new0  RConnTagsString=__new0  BranchType=R  Resistance=1e6  Inductance=1e-3  SetiL0=off  InitialCurrent=0  Capacitance=1e-6  Setx0=off  InitialVoltage=0  Measurements=None
      settings: SourceProductName=Simscape Electrical
  meas cur2 : powerlib/Measurements/Current Measurement  PhasorSimulation=on  OutputType=Complex  PSBequivalent=0
      settings: SourceProductName=Simscape Electrical
  Conn1 : PMIOPort  Side=Left
  Conn2 : PMIOPort  Port=2  Side=Right
  Out1 : Outport
  wires:
  meas cur2/1 -> Out1/1
  Clock/1 -> Load Data 1-D Lookup Table/1
  Magnitude-Angle to Complex1/1 -> Controlled Current Source4/1
  Load Data 1-D Lookup Table/1 -> Gain6/1
  Complex to Magnitude-Angle/1 -> Magnitude-Angle to Complex1/2
  Gain10/1 -> Magnitude-Angle to Complex1/1
  Gain6/1 -> Gain10/1
  [Vsec] -> Complex to Magnitude-Angle/1
  connections:
  Controlled Current Source4/LConn1 -- Conn2/RConn1 -- Snubber3/RConn1
  Controlled Current Source4/RConn1 -- meas cur2/RConn1 -- Snubber3/LConn1
  Conn1/RConn1 -- meas cur2/LConn1

== system power_microgrid_v5_battery/House 34 ==
  Clock : Clock
  Complex to Magnitude-Angle : ComplexToMagnitudeAngle  Output=Angle
  Controlled Current Source4 : powerlib/Electrical Sources/Controlled Current Source  Initialize=on  Source_Type=AC  Amplitude=0  Phase=0  Frequency=50  Measurements=None
      settings: SourceProductName=Simscape Electrical
  Gain10 : Gain  Gain=sqrt(2)
  Gain6 : Gain  Gain=-1/230
  Load Data 1-D Lookup Table : Lookup_n-D  NumberOfTableDimensions=1  BreakpointsForDimension1="[0.00\t600.00\t1200.00\t1800.00\t2400.00\t3000.00\t3600.00\t4200.00\t4800.00\t5400.00\t6000.00\t6600.00\t7200.00\t7800.00\t8400.00\t9000.00\t9600.00\t10200.00\t10800.00\t11400.00\t12000.00\t12600.00\t13200.00\t13800.00\t14400.00\t15000.00\t15600.00\t16200.00\t16800.00\t17400.00\t18000.00\t18600.00\t19200.00\t19800.00\t20400.00\t21000.00\t21600.00\t22200.00\t22800.00\t23400.00\t24000.00\t24600.00\t25200.00\t25800.00\t26400.00\t27000.00\t27600.00\t28200.00\t28800.00\t29400.00\t30000.00\t30600.00\t31200.00\t31800.00\t32400.00\t33000.00\t33600.00\t34200.00\t34800.00\t35400.00\t36000.00\t36600.00\t37200.00\t37800.00\t38400.00\t39000.00\t39600.00\t40200.00\t40800.00\t41400.00\t42000.00\t42600.00\t43200.00\t43800.00\t44400.00\t45000.00\t45600.00\t46200.00\t46800.00\t47400.00\t48000.00\t48600.00\t49200.00\t49800.00\t50400.00\t51000.00\t51600.00\t52200.00\t52800.00\t53400.00\t54000.00\t54600.00\t55200.00\t55800.00\t56400.00\t57000.00\t57600.00\t58200.00\t58800.00\t59400.00\t60000.00\t60600.00\t61200.00\t61800.00\t62400.00\t63000.00\t63600.00\t64200.00\t64800.00\t65400.00\t66000.00\t66600.00\t67200.00\t67800.00\t68400.00\t69000.00\t69600.00\t70200.00\t70800.00\t71400.00\t72000.00\t72600.00\t73200.00\t73800.00\t74400.00\t75000.00\t75600.00\t76200.00\t76800.00\t77400.00\t78000.00\t78600.00\t79200.00\t79800.00\t80400.00\t81000.00\t81600.00\t82200.00\t82800.00\t83400.00\t84000.00\t84600.00\t85200.00\t85800.00\t86400.00]"  BeginIndexSearchUsingPreviousIndexResult=on  Table="[1249.6\t1321.5\t1264.8\t1197.8\t636.4\t449.7\t418.3\t382.3\t388.2\t394.0\t381.4\t352.7\t307.3\t261.7\t214.1\t200.0\t192.7\t201.8\t200.7\t195.8\t196.0\t199.1\t204.7\t193.8\t179.3\t190.3\t190.0\t193.3\t191.8\t187.4\t181.3\t191.8\t193.1\t186.4\t206.3\t215.8\t201.0\t258.4\t233.1\t239.4\t245.9\t279.3\t328.0\t478.8\t590.9\t623.2\t711.5\t731.6\t817.3\t846.6\t980.1\t816.5\t947.4\t949.3\t1082.2\t873.2\t930.4\t882.0\t855.7\t823.6\t788.1\t836.4\t796.1\t819.8\t851.2\t875.5\t798.5\t729.9\t728.8\t746.0\t634.5\t627.5\t716.5\t796.0\t804.6\t896.9\t925.6\t965.5\t887.1\t813.0\t859.8\t799.0\t838.9\t776.1\t746.4\t744.2\t744.4\t742.2\t764.7\t806.9\t796.9\t694.1\t689.4\t616.7\t637.9\t686.7\t746.7\t770.0\t816.1\t900.2\t1025.9\t1030.1\t1143.1\t1112.0\t1121.9\t1260.6\t1220.7\t1254.0\t1246.8\t1243.4\t1158.2\t1113.4\t1233.0\t1187.3\t1279.1\t1251.7\t1285.1\t1265.1\t1329.1\t1371.9\t1396.5\t1367.7\t1278.2\t1308.3\t1269.3\t1234.1\t1170.5\t1120.3\t1111.6\t1182.3\t1082.0\t1034.8\t1033.4\t952.5\t934.7\t842.2\t1302.8\t1459.0\t1469.8\t1449.8\t1432.7\t1428.8\t1360.5\t1299.8\t1249.6]"  InternalRulePriority=Speed  RndMeth=Simplest  InputSameDT=on
  Magnitude-Angle to Complex1 : MagnitudeAngleToComplex
  Snubber3 : powerlib/Elements/Series RLC Branch  LConnTagsString=__new0  RConnTagsString=__new0  BranchType=R  Resistance=1e6  Inductance=1e-3  SetiL0=off  InitialCurrent=0  Capacitance=1e-6  Setx0=off  InitialVoltage=0  Measurements=None
      settings: SourceProductName=Simscape Electrical
  meas cur2 : powerlib/Measurements/Current Measurement  PhasorSimulation=on  OutputType=Complex  PSBequivalent=0
      settings: SourceProductName=Simscape Electrical
  Conn1 : PMIOPort  Side=Left
  Conn2 : PMIOPort  Port=2  Side=Right
  Out1 : Outport
  wires:
  meas cur2/1 -> Out1/1
  Clock/1 -> Load Data 1-D Lookup Table/1
  Magnitude-Angle to Complex1/1 -> Controlled Current Source4/1
  Load Data 1-D Lookup Table/1 -> Gain6/1
  Complex to Magnitude-Angle/1 -> Magnitude-Angle to Complex1/2
  Gain10/1 -> Magnitude-Angle to Complex1/1
  Gain6/1 -> Gain10/1
  [Vsec] -> Complex to Magnitude-Angle/1
  connections:
  Conn1/RConn1 -- meas cur2/LConn1
  Snubber3/LConn1 -- meas cur2/RConn1 -- Controlled Current Source4/RConn1
  Snubber3/RConn1 -- Controlled Current Source4/LConn1 -- Conn2/RConn1

== system power_microgrid_v5_battery/House 35 ==
  Clock : Clock
  Complex to Magnitude-Angle : ComplexToMagnitudeAngle  Output=Angle
  Controlled Current Source4 : powerlib/Electrical Sources/Controlled Current Source  Initialize=on  Source_Type=AC  Amplitude=0  Phase=0  Frequency=50  Measurements=None
      settings: SourceProductName=Simscape Electrical
  Gain10 : Gain  Gain=sqrt(2)
  Gain6 : Gain  Gain=-1/230
  Load Data 1-D Lookup Table : Lookup_n-D  NumberOfTableDimensions=1  BreakpointsForDimension1="[0.00\t600.00\t1200.00\t1800.00\t2400.00\t3000.00\t3600.00\t4200.00\t4800.00\t5400.00\t6000.00\t6600.00\t7200.00\t7800.00\t8400.00\t9000.00\t9600.00\t10200.00\t10800.00\t11400.00\t12000.00\t12600.00\t13200.00\t13800.00\t14400.00\t15000.00\t15600.00\t16200.00\t16800.00\t17400.00\t18000.00\t18600.00\t19200.00\t19800.00\t20400.00\t21000.00\t21600.00\t22200.00\t22800.00\t23400.00\t24000.00\t24600.00\t25200.00\t25800.00\t26400.00\t27000.00\t27600.00\t28200.00\t28800.00\t29400.00\t30000.00\t30600.00\t31200.00\t31800.00\t32400.00\t33000.00\t33600.00\t34200.00\t34800.00\t35400.00\t36000.00\t36600.00\t37200.00\t37800.00\t38400.00\t39000.00\t39600.00\t40200.00\t40800.00\t41400.00\t42000.00\t42600.00\t43200.00\t43800.00\t44400.00\t45000.00\t45600.00\t46200.00\t46800.00\t47400.00\t48000.00\t48600.00\t49200.00\t49800.00\t50400.00\t51000.00\t51600.00\t52200.00\t52800.00\t53400.00\t54000.00\t54600.00\t55200.00\t55800.00\t56400.00\t57000.00\t57600.00\t58200.00\t58800.00\t59400.00\t60000.00\t60600.00\t61200.00\t61800.00\t62400.00\t63000.00\t63600.00\t64200.00\t64800.00\t65400.00\t66000.00\t66600.00\t67200.00\t67800.00\t68400.00\t69000.00\t69600.00\t70200.00\t70800.00\t71400.00\t72000.00\t72600.00\t73200.00\t73800.00\t74400.00\t75000.00\t75600.00\t76200.00\t76800.00\t77400.00\t78000.00\t78600.00\t79200.00\t79800.00\t80400.00\t81000.00\t81600.00\t82200.00\t82800.00\t83400.00\t84000.00\t84600.00\t85200.00\t85800.00\t86400.00]"  BeginIndexSearchUsingPreviousIndexResult=on  Table="[1249.6\t1321.5\t1264.8\t1197.8\t636.4\t449.7\t418.3\t382.3\t388.2\t394.0\t381.4\t352.7\t307.3\t261.7\t214.1\t200.0\t192.7\t201.8\t200.7\t195.8\t196.0\t199.1\t204.7\t193.8\t179.3\t190.3\t190.0\t193.3\t191.8\t187.4\t181.3\t191.8\t193.1\t186.4\t206.3\t215.8\t201.0\t258.4\t233.1\t239.4\t245.9\t279.3\t328.0\t478.8\t590.9\t623.2\t711.5\t731.6\t817.3\t846.6\t980.1\t816.5\t947.4\t949.3\t1082.2\t873.2\t930.4\t882.0\t855.7\t823.6\t788.1\t836.4\t796.1\t819.8\t851.2\t875.5\t798.5\t729.9\t728.8\t746.0\t634.5\t627.5\t716.5\t796.0\t804.6\t896.9\t925.6\t965.5\t887.1\t813.0\t859.8\t799.0\t838.9\t776.1\t746.4\t744.2\t744.4\t742.2\t764.7\t806.9\t796.9\t694.1\t689.4\t616.7\t637.9\t686.7\t746.7\t770.0\t816.1\t900.2\t1025.9\t1030.1\t1143.1\t1112.0\t1121.9\t1260.6\t1220.7\t1254.0\t1246.8\t1243.4\t1158.2\t1113.4\t1233.0\t1187.3\t1279.1\t1251.7\t1285.1\t1265.1\t1329.1\t1371.9\t1396.5\t1367.7\t1278.2\t1308.3\t1269.3\t1234.1\t1170.5\t1120.3\t1111.6\t1182.3\t1082.0\t1034.8\t1033.4\t952.5\t934.7\t842.2\t1302.8\t1459.0\t1469.8\t1449.8\t1432.7\t1428.8\t1360.5\t1299.8\t1249.6]"  InternalRulePriority=Speed  RndMeth=Simplest  InputSameDT=on
  Magnitude-Angle to Complex1 : MagnitudeAngleToComplex
  Snubber3 : powerlib/Elements/Series RLC Branch  LConnTagsString=__new0  RConnTagsString=__new0  BranchType=R  Resistance=1e6  Inductance=1e-3  SetiL0=off  InitialCurrent=0  Capacitance=1e-6  Setx0=off  InitialVoltage=0  Measurements=None
      settings: SourceProductName=Simscape Electrical
  meas cur2 : powerlib/Measurements/Current Measurement  PhasorSimulation=on  OutputType=Complex  PSBequivalent=0
      settings: SourceProductName=Simscape Electrical
  Conn1 : PMIOPort  Side=Left
  Conn2 : PMIOPort  Port=2  Side=Right
  Out1 : Outport
  wires:
  Magnitude-Angle to Complex1/1 -> Controlled Current Source4/1
  meas cur2/1 -> Out1/1
  Clock/1 -> Load Data 1-D Lookup Table/1
  Load Data 1-D Lookup Table/1 -> Gain6/1
  [Vsec] -> Complex to Magnitude-Angle/1
  Gain6/1 -> Gain10/1
  Gain10/1 -> Magnitude-Angle to Complex1/1
  Complex to Magnitude-Angle/1 -> Magnitude-Angle to Complex1/2
  connections:
  meas cur2/LConn1 -- Conn1/RConn1
  Snubber3/LConn1 -- Controlled Current Source4/RConn1 -- meas cur2/RConn1
  Snubber3/RConn1 -- Controlled Current Source4/LConn1 -- Conn2/RConn1

== system power_microgrid_v5_battery/House 36 ==
  Clock : Clock
  Complex to Magnitude-Angle : ComplexToMagnitudeAngle  Output=Angle
  Controlled Current Source4 : powerlib/Electrical Sources/Controlled Current Source  Initialize=on  Source_Type=AC  Amplitude=0  Phase=0  Frequency=50  Measurements=None
      settings: SourceProductName=Simscape Electrical
  Gain10 : Gain  Gain=sqrt(2)
  Gain6 : Gain  Gain=-1/230
  Load Data 1-D Lookup Table : Lookup_n-D  NumberOfTableDimensions=1  BreakpointsForDimension1="[0.00\t600.00\t1200.00\t1800.00\t2400.00\t3000.00\t3600.00\t4200.00\t4800.00\t5400.00\t6000.00\t6600.00\t7200.00\t7800.00\t8400.00\t9000.00\t9600.00\t10200.00\t10800.00\t11400.00\t12000.00\t12600.00\t13200.00\t13800.00\t14400.00\t15000.00\t15600.00\t16200.00\t16800.00\t17400.00\t18000.00\t18600.00\t19200.00\t19800.00\t20400.00\t21000.00\t21600.00\t22200.00\t22800.00\t23400.00\t24000.00\t24600.00\t25200.00\t25800.00\t26400.00\t27000.00\t27600.00\t28200.00\t28800.00\t29400.00\t30000.00\t30600.00\t31200.00\t31800.00\t32400.00\t33000.00\t33600.00\t34200.00\t34800.00\t35400.00\t36000.00\t36600.00\t37200.00\t37800.00\t38400.00\t39000.00\t39600.00\t40200.00\t40800.00\t41400.00\t42000.00\t42600.00\t43200.00\t43800.00\t44400.00\t45000.00\t45600.00\t46200.00\t46800.00\t47400.00\t48000.00\t48600.00\t49200.00\t49800.00\t50400.00\t51000.00\t51600.00\t52200.00\t52800.00\t53400.00\t54000.00\t54600.00\t55200.00\t55800.00\t56400.00\t57000.00\t57600.00\t58200.00\t58800.00\t59400.00\t60000.00\t60600.00\t61200.00\t61800.00\t62400.00\t63000.00\t63600.00\t64200.00\t64800.00\t65400.00\t66000.00\t66600.00\t67200.00\t67800.00\t68400.00\t69000.00\t69600.00\t70200.00\t70800.00\t71400.00\t72000.00\t72600.00\t73200.00\t73800.00\t74400.00\t75000.00\t75600.00\t76200.00\t76800.00\t77400.00\t78000.00\t78600.00\t79200.00\t79800.00\t80400.00\t81000.00\t81600.00\t82200.00\t82800.00\t83400.00\t84000.00\t84600.00\t85200.00\t85800.00\t86400.00]"  BeginIndexSearchUsingPreviousIndexResult=on  Table="[287.9\t293.8\t263.0\t241.1\t234.1\t222.8\t214.5\t212.4\t211.1\t207.7\t200.9\t198.4\t194.4\t188.2\t185.8\t183.7\t189.6\t185.1\t179.0\t187.6\t179.7\t177.3\t169.0\t173.0\t169.3\t171.8\t165.9\t166.7\t170.5\t173.6\t179.5\t181.7\t196.2\t192.2\t177.7\t185.2\t250.8\t216.4\t218.6\t232.6\t256.0\t271.2\t292.1\t313.3\t326.6\t375.3\t421.6\t371.9\t375.5\t386.5\t395.4\t389.8\t364.4\t413.6\t395.4\t408.4\t410.4\t379.8\t364.2\t381.0\t383.4\t378.7\t384.3\t387.0\t365.1\t363.6\t369.7\t354.4\t367.8\t353.9\t361.0\t349.4\t377.3\t400.1\t383.7\t374.8\t382.5\t353.8\t359.6\t363.7\t347.9\t331.7\t346.5\t345.9\t334.7\t324.2\t332.7\t349.6\t363.2\t345.4\t350.9\t355.6\t374.0\t393.2\t389.1\t383.8\t404.1\t426.3\t443.7\t449.0\t452.4\t452.9\t477.6\t496.2\t496.4\t518.8\t529.6\t538.5\t545.1\t587.6\t591.8\t593.3\t586.6\t595.1\t603.6\t621.9\t603.6\t607.2\t582.9\t601.9\t605.1\t579.6\t566.2\t557.6\t554.0\t551.3\t552.4\t585.1\t576.4\t564.1\t559.0\t553.1\t536.3\t517.7\t521.5\t519.5\t485.4\t437.7\t418.5\t395.9\t370.8\t353.7\t336.4\t311.0\t287.9]"  InternalRulePriority=Speed  RndMeth=Simplest  InputSameDT=on
  Magnitude-Angle to Complex1 : MagnitudeAngleToComplex
  Snubber3 : powerlib/Elements/Series RLC Branch  LConnTagsString=__new0  RConnTagsString=__new0  BranchType=R  Resistance=1e6  Inductance=1e-3  SetiL0=off  InitialCurrent=0  Capacitance=1e-6  Setx0=off  InitialVoltage=0  Measurements=None
      settings: SourceProductName=Simscape Electrical
  meas cur2 : powerlib/Measurements/Current Measurement  PhasorSimulation=on  OutputType=Complex  PSBequivalent=0
      settings: SourceProductName=Simscape Electrical
  Conn1 : PMIOPort  Side=Left
  Conn2 : PMIOPort  Port=2  Side=Right
  Out1 : Outport
  wires:
  meas cur2/1 -> Out1/1
  Clock/1 -> Load Data 1-D Lookup Table/1
  Magnitude-Angle to Complex1/1 -> Controlled Current Source4/1
  Load Data 1-D Lookup Table/1 -> Gain6/1
  Complex to Magnitude-Angle/1 -> Magnitude-Angle to Complex1/2
  Gain10/1 -> Magnitude-Angle to Complex1/1
  Gain6/1 -> Gain10/1
  [Vsec] -> Complex to Magnitude-Angle/1
  connections:
  Controlled Current Source4/LConn1 -- Conn2/RConn1 -- Snubber3/RConn1
  Controlled Current Source4/RConn1 -- meas cur2/RConn1 -- Snubber3/LConn1
  Conn1/RConn1 -- meas cur2/LConn1
